simulink model "kalman_filter_dynamic"  (R2024b)
settings: Solver=VariableStepAuto  StartTime=0.0  StopTime=10.0  RelTol=1e-3
settings Model: Creator=aakas  LastModifiedBy=aakas

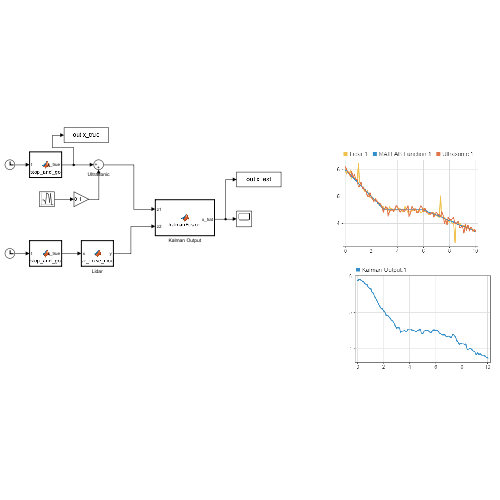
[thumbnail: Simulink's stored preview of the top-level diagram]
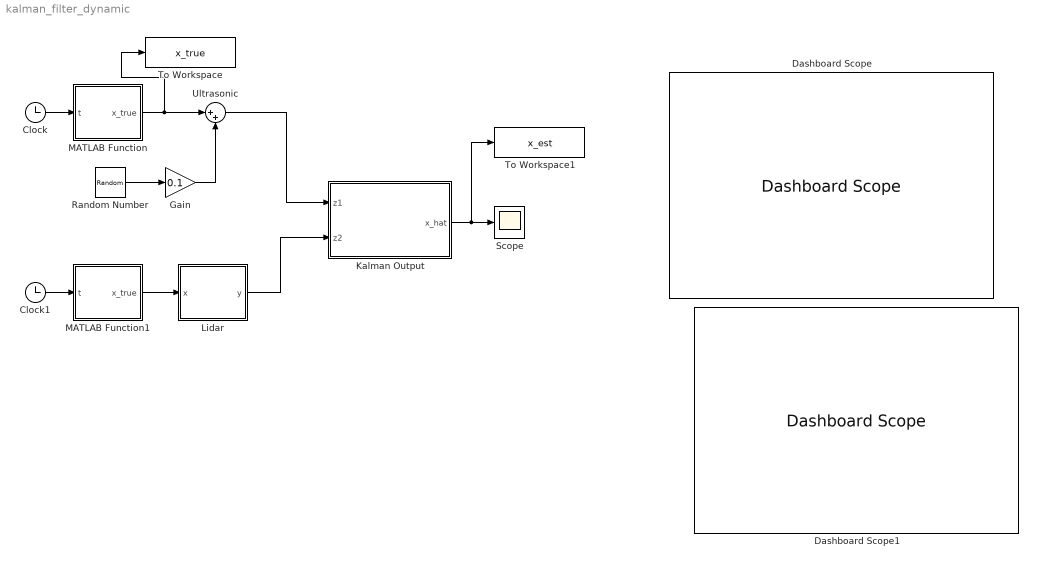
== system kalman_filter_dynamic ==
  Clock : Clock
  Clock1 : Clock
  Dashboard Scope : DashboardScope
  Dashboard Scope1 : DashboardScope
  Gain : Gain  Gain=0.1
  Kalman Output : MATLAB Function  TreatAsAtomicUnit=on
  Lidar : MATLAB Function  TreatAsAtomicUnit=on
  MATLAB Function : MATLAB Function  TreatAsAtomicUnit=on
  MATLAB Function1 : MATLAB Function  TreatAsAtomicUnit=on
  Random Number : RandomNumber  SampleTime=0.1
  Scope : Scope
  To Workspace : ToWorkspace  VariableName=x_true  SaveFormat=Timeseries  SampleTime=-1
  To Workspace1 : ToWorkspace  VariableName=x_est  SaveFormat=Timeseries  SampleTime=-1
  Ultrasonic : Sum  Inputs=|++
  wires:
  Clock/1 -> MATLAB Function/1(t)
  Random Number/1 -> Gain/1
  Gain/1 -> Ultrasonic/2
  MATLAB Function/1(x_true) -> To Workspace/1, Ultrasonic/1
  Clock1/1 -> MATLAB Function1/1(t)
  MATLAB Function1/1(x_true) -> Lidar/1(x)
  Lidar/1(y) -> Kalman Output/2(z2)
  Ultrasonic/1 -> Kalman Output/1(z1)
  Kalman Output/1(x_hat) -> To Workspace1/1, Scope/1

== matlab function kalman_filter_dynamic/MATLAB Function ==
  data: x_true output; t input
function x_true = stop_and_go(t)

if t < 3
    x_true = 6 - 0.5 * t;
elseif t < 6
    x_true = 4.5;
else
    x_true = 4.5 - 0.2 * (t - 6);
end

== matlab function kalman_filter_dynamic/Lidar ==
  data: y output; x input
function y = lidar_noise_model(x)
% x: true distance
% y: noisy LiDAR reading

% Add small Gaussian noise
noise = 0.05 * randn();

% Random spike (5% chance)
if rand() < 0.05
    spike = 2 * (rand() - 0.5);  % Random spike between -1 and 1
else
    spike = 0;
end

y = x + noise + spike;

== matlab function kalman_filter_dynamic/Kalman Output ==
  data: x_hat output; z1 input; z2 input
function x_hat = kalmanFusion(z1, z2)

%#codegen

persistent x P Q R1 R2 H I

if isempty(x)
    x = 0;                      % Initial estimate
    P = 1;                      % Initial error covariance
    Q = 0.01;                   % Process noise
    R1 = 0.05;                  % LiDAR noise
    R2 = 0.1;                   % Ultrasonic noise
    H = 1;                      % Measurement model
    I = 1;                      % Identity matrix
end

% Measurement fusion (simple average or weighted)
z = (z1/R1 + z2/R2) / (1/R1 + 1/R2);
R = 1 / (1/R1 + 1/R2);  % Combined measurement noise

% Prediction
x_pred = x;
P_pred = P + Q;

% Update
K = P_pred * H / (H * P_pred * H + R);  % Kalman Gain
x = x_pred + K * (z - H * x_pred);
P = (I - K * H) * P_pred;

x_hat = x;

== matlab function kalman_filter_dynamic/MATLAB Function1 ==
  data: x_true output; t input
function x_true = stop_and_go(t)
%#codegen

if t < 3
    x_true = 6 - 0.5 * t;
elseif t < 6
    x_true = 4.5; % stopped
else
    x_true = 4.5 - 0.2 * (t - 6);
end
